simulink model "BlocoHidraulico"  (R2025a)
settings: Solver=ode15s  StartTime=0.0  StopTime=4  MaxStep=1e-4  RelTol=1e-3
values from neighbouring files (symbols this model uses):
  Pret = 1e5    (= 100000)    [ensaio_integrado_malha_aberta_real.m]    (also in ensaio_malha_fechada_lqi.m)
  Psup0 = Pret    (= 100000)    [ensaio_integrado_malha_aberta_real.m]
  Pw0 = Pret    (= 100000)    [ensaio_integrado_malha_aberta_real.m]
settings Model: Creator=uidq5744  LastModifiedBy=uidq5744

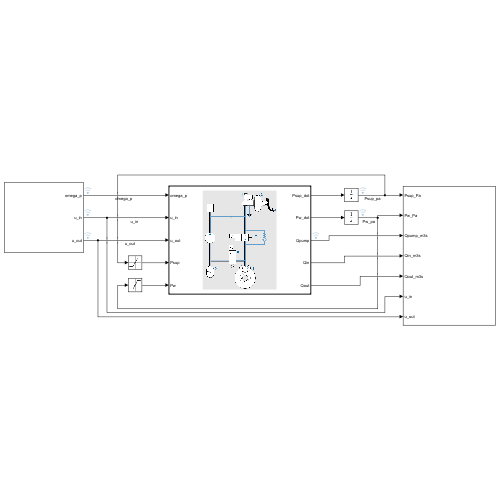
[thumbnail: Simulink's stored preview of the top-level diagram]
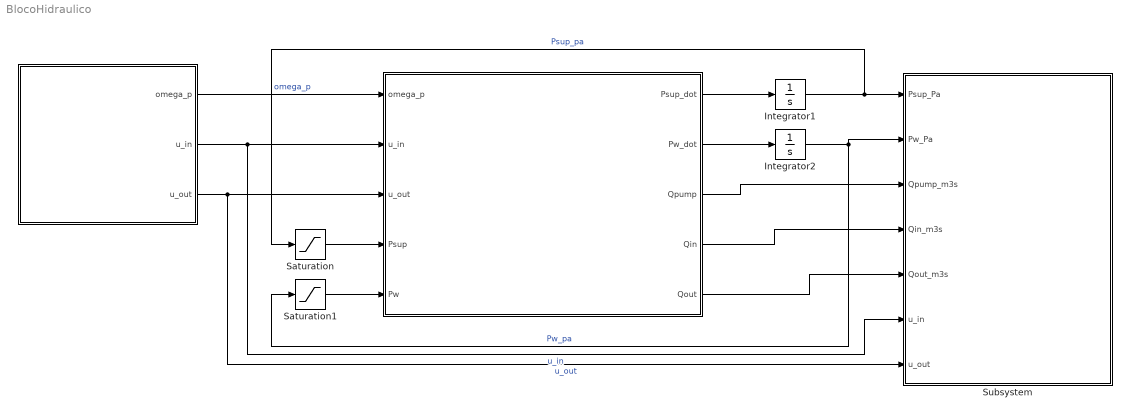
== system BlocoHidraulico ==
  " " : Subsystem
  "  " : MATLAB Function  TreatAsAtomicUnit=on
  Integrator1 : Integrator  InitialCondition=Psup0
  Integrator2 : Integrator  InitialCondition=Pw0
  Saturation : Saturate  UpperLimit=2.5e7  LowerLimit=Pret
  Saturation1 : Saturate  UpperLimit=2.5e7  LowerLimit=Pret
  Subsystem : Subsystem
  wires:
  Integrator1/1 -> Saturation/1, Subsystem/1(Psup_Pa)  "Psup_pa"
  " "/1(omega_p) -> "  "/1(omega_p)  "omega_p"
  " "/2(u_in) -> "  "/2(u_in), Subsystem/6(u_in)  "u_in"
  " "/3(u_out) -> "  "/3(u_out), Subsystem/7(u_out)  "u_out"
  "  "/1(Psup_dot) -> Integrator1/1
  "  "/2(Pw_dot) -> Integrator2/1
  Integrator2/1 -> Saturation1/1, Subsystem/2(Pw_Pa)  "Pw_pa"
  Saturation/1 -> "  "/4(Psup)
  Saturation1/1 -> "  "/5(Pw)
  "  "/3(Qpump) -> Subsystem/3(Qpump_m3s)
  "  "/4(Qin) -> Subsystem/4(Qin_m3s)
  "  "/5(Qout) -> Subsystem/5(Qout_m3s)

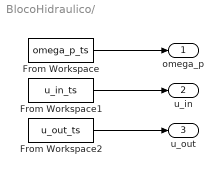
== system BlocoHidraulico/  ==
  From Workspace : FromWorkspace  VariableName=omega_p_ts
  From Workspace1 : FromWorkspace  VariableName=u_in_ts
  From Workspace2 : FromWorkspace  VariableName=u_out_ts
  omega_p : Outport
  u_in : Outport  Port=2
  u_out : Outport  Port=3
  wires:
  From Workspace/1 -> omega_p/1
  From Workspace1/1 -> u_in/1
  From Workspace2/1 -> u_out/1

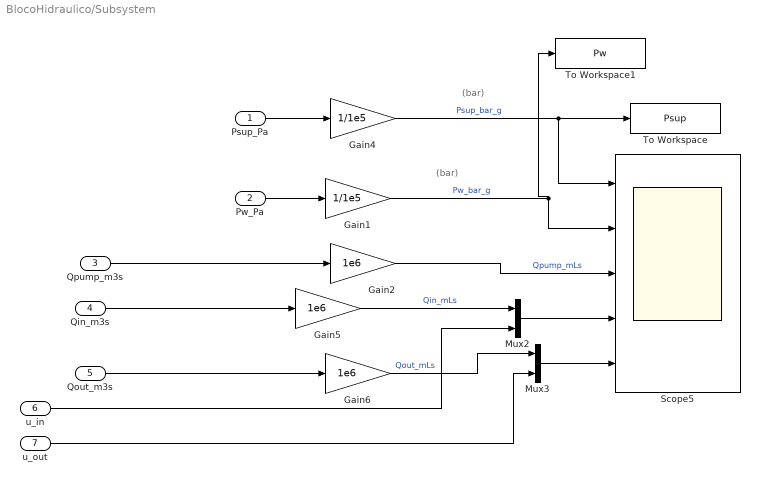
== system BlocoHidraulico/Subsystem ==
  note: (bar)
  note: (bar)
  Psup_Pa : Inport
  Pw_Pa : Inport  Port=2
  Qpump_m3s : Inport  Port=3
  Qin_m3s : Inport  Port=4
  Qout_m3s : Inport  Port=5
  u_in : Inport  Port=6
  u_out : Inport  Port=7
  Gain1 : Gain  Gain=1/1e5
  Gain2 : Gain  Gain=1e6
  Gain4 : Gain  Gain=1/1e5
  Gain5 : Gain  Gain=1e6
  Gain6 : Gain  Gain=1e6
  Mux2 : Mux  Inputs=2
  Mux3 : Mux  Inputs=2
  Scope5 : Scope  NumInputPorts=5
      settings: ActiveDisplayYMinimum=-13.920770076157355  ActiveDisplayYMaximum=135.28693068541622  DataLoggingVariableName=ScopeData6
  To Workspace : ToWorkspace  VariableName=Psup  SaveFormat=Timeseries  SampleTime=-1
  To Workspace1 : ToWorkspace  VariableName=Pw  SaveFormat=Timeseries  SampleTime=-1
  wires:
  Gain1/1 -> Scope5/2, To Workspace1/1  "Pw_bar_g"
  Mux2/1 -> Scope5/4
  Gain5/1 -> Mux2/1  "Qin_mLs"
  u_in/1 -> Mux2/2
  Gain2/1 -> Scope5/3  "Qpump_mLs"
  Gain4/1 -> Scope5/1, To Workspace/1  "Psup_bar_g"
  Gain6/1 -> Mux3/1  "Qout_mLs"
  Mux3/1 -> Scope5/5
  Psup_Pa/1 -> Gain4/1
  Qpump_m3s/1 -> Gain2/1
  Qout_m3s/1 -> Gain6/1
  Qin_m3s/1 -> Gain5/1
  u_out/1 -> Mux3/2
  Pw_Pa/1 -> Gain1/1

== matlab function BlocoHidraulico/   ==
  data: omega_p input; Psup_dot output; u_in input; u_out input; Psup input; Pw input; Pw_dot output; Qpump output; Qin output; Qout output
function [Psup_dot, Pw_dot, Qpump, Qin, Qout] = Bloco_Hidraulico_2P(omega_p, u_in, u_out, Psup, Pw)
% omega_p: rad/s (>=0)
% u_in, u_out: 0..1 (PWM normalizado / abertura proporcional)
% Psup, Pw: Pa
% Saídas: derivadas de pressão e vazões (m^3/s)

% ---------- parâmetros hidráulicos básicos ----------
beta = 1.5e9;   % Pa - módulo volumétrico efetivo (óleo + mangueiras)
rho  = 850;     % kg/m^3 - densidade típica de fluido de freio
Pret = 1e5;     % Pa - pressão de retorno (aprox. atmosférica)

% ---------- volumes efetivos ----------
% Ordens de grandeza compatíveis com circuitos de freio/HCU:
% - Lv2014, ChenLv2017: pequenas câmaras, respostas de 80–300 MPa/s.
%
% Vsup: volume efetivo do manifold/suprimento (linha de alta + câmara da HCU)
% Vw  : volume efetivo do circuito "roda"/caliper (câmara da pinça + linha)
Vsup = 6.0e-5;   % m^3  (~100 mL)
Vw   = 1.0e-5;   % m^3  (~10 mL)

% ---------- bomba (modelo linear simples) ----------
% Referência: bombas de HCU/IEB com deslocamentos da ordem de 0.1–1 cm^3/volta,
% vazões < 1 L/min em regimes típicos (WangBingbing2015, MotorParametricDesign2023).
%
Dp_rev = 5e-7;           % m^3/rev (0.5 cm^3/1000 rev; pequeno deslocamento por volta)
Nv     = 0.85;           % eficiência volumétrica
Kb     = Nv * (Dp_rev/(2*pi));   % m^3/rad  (Qpump = Kb*omega_p)
Klb    = 6.8e-13;          % (m^3/s)/Pa - vazamento interno equivalente (3e-13 a 8e-13)
% Klb (vazamento/bypass interno “de verdade”): 1e-14 a 5e-13 (ordem menor que hoje)

% ---------- válvulas (lei do orifício) ----------
% Coerente com diâmetros de ~0.6–0.8 mm (ChenLv2017, ProportionalPressureABS2023):
% A = pi*(d/2)^2. Para d ≈ 0.7 mm -> A ≈ 3.8e-7 m^2.
% Usamos área máxima ligeiramente menor para representar abertura efetiva.
Cv_in   = 0.62;          % coeficiente de descarga típico
Cv_out  = 0.62;
Ain_max = 3.0e-7;        % m^2 - área máx. da válvula de entrada
Aout_max= 3.0e-7;        % m^2 - área máx. da válvula de saída

% Vazamentos opcionais (para estabilidade numérica / perdas pequenas)
Kleak_sup = 0;           % (m^3/s)/Pa
Kleak_w   = 0;           % (m^3/s)/Pa

% ---------- sanitização de entradas ----------
if omega_p < 0
    omega_p = 0;
end
u_in  = min(max(u_in,  0), 1);
u_out = min(max(u_out, 0), 1);

% Evita pressões abaixo do retorno (numérico)
Psup = max(Psup, Pret);
Pw   = max(Pw,   Pret);

% ---------- bomba -> suprimento ----------
Qpump = Kb*omega_p - Klb*(Psup - Pret);
% Nota: usa (Psup - Pret) para não "puxar" abaixo da pressão de retorno.

% ---------- suprimento -> roda (válvula de entrada) ----------
dPin = max(Psup - Pw, 0);
Qin  = Cv_in * (Ain_max * u_in) * sqrt(2*dPin/rho);

% ---------- roda -> retorno (válvula de saída) ----------
dPout = max(Pw - Pret, 0);
Qout  = Cv_out * (Aout_max * u_out) * sqrt(2*dPout/rho);

% ---------- dinâmica das pressões ----------
Psup_dot = (beta/Vsup) * ( Qpump - Qin - Kleak_sup*(Psup - Pret) );
Pw_dot   = (beta/Vw)   * ( Qin - Qout - Kleak_w*(Pw   - Pret) );
end

%%
% β e ρ mantidos (compatíveis com Lv2014, MotorParametricDesign2023).
% Volumes Vsup, Vw ajustados para ordens de 10⁻⁶–10⁻⁷ m³ (câmara pequena de HCU e cilindro de roda) coerentes com Lv2014 / ChenLv2017 / ZengYangHuang2023.
% Bomba dimensionada para vazões ~0.5–1 L/min em faixas de rpm típicas de bomba ESC (coerente com MotorParametricDesign2023 e WangBingbing2015).
% Áreas de válvulas baseadas em diâmetros ~0.6–0.8 mm (ProportionalPressureABS2023, ChenLv2017).

% Com Vsup ≈ 2 mL e Vw ≈ 0.5 mL, beta/V fica na ordem de 10¹⁴–10¹⁵ s⁻¹·m⁻³, o que, combinado com vazões de ~10⁻⁶–10⁻⁵ m³/s, gera dP/dt na faixa de dezenas a poucas centenas de MPa/s – alinhado com os ~88.8 MPa/s (subida) e ~324.9 MPa/s (descida) medidos em ZengYangHuang2023.
% As áreas de válvula (~3e-7 m²) correspondem a diâmetros ~0.6–0.7 mm, compatíveis com os assentos/agulhas dos artigos ChenLv2017 e ProportionalPressureABS2023.
% O deslocamento da bomba (5e-7 m³/rev) é conservador, mas suficiente para gerar pressões de alguns MPa em tempos da ordem de 0.1–0.2 s para testes de malha aberta.


% function [Psup_dot, Pw_dot, Qpump, Qin, Qout] = Bloco_Hidraulico_2P(omega_p, u_in, u_out, Psup, Pw)
% % omega_p: rad/s (>=0)
% % u_in, u_out: 0..1 (PWM normalizado)
% % Psup, Pw: Pa
% % Saídas: derivadas de pressão e vazões (m^3/s)
% 
% % ---------- parâmetros ----------
% beta   = 1.5e9;      % Pa (módulo volumétrico efetivo)
% rho    = 850;        % kg/m^3
% Pret   = 1e5;        % Pa (reservatório/retorno)
% 
% % Volume teorico
% % Vsup   = 2.0e-5;     % m^3  (volume efetivo do manifold/suprimento) AJUSTAR
% % Vw     = 1.0e-5;     % m^3  (volume efetivo do circuito "roda"/caliper) AJUSTAR
% 
% % Volumes reduzidos (faixa de pressao mais alta)
% Vsup   = 5.0e-7;     % m^3  (volume efetivo do manifold/suprimento)
% Vw     = 5.0e-8;     % m^3  (volume efetivo do circuito "roda"/caliper)
% 
% % % Bomba (modelo linear simples)
% % Dp_rev = 1e-6;       % m^3/rev
% % Nv  = 0.85;       % Eficiência volumétrica da bomba
% % Kb     = Nv*(Dp_rev/(2*pi)); % m^3/rad
% % Klb    = 1e-10;      % (m^3/s)/Pa  (vazamento interno equivalente)
% 
% % Bomba (parâmetros ajustados)
% Dp_rev = 1e-5;       % m^3/rev (deslocamento volumétrico por volta)
% Nv     = 0.85;       % Eficiência volumétrica da bomba
% Kb     = Nv*(Dp_rev/(2*pi)); % m^3/rad
% Klb    = 1e-11;      % (m^3/s)/Pa  (vazamento interno equivalente)
% 
% % Válvulas (lei do orifício)
% Cv_in   = 0.62;
% Cv_out  = 0.62;
% Ain_max = 1e-7;      % m^2
% Aout_max= 1e-7;      % m^2
% 
% Kleak_sup = 0;       % (m^3/s)/Pa opcional
% Kleak_w   = 0;       % (m^3/s)/Pa opcional
% 
% % ---------- sanitização ----------
% if omega_p < 0, omega_p = 0; end
% u_in  = min(max(u_in, 0), 1);
% u_out = min(max(u_out,0), 1);
% 
% % Evita pressões abaixo do retorno (numérico)
% Psup = max(Psup, Pret);
% Pw   = max(Pw,   Pret);
% 
% % ---------- bomba -> suprimento ----------
% Qpump = Kb*omega_p - Klb*(Psup - Pret);
% % Observação: use (Psup-Pret) aqui pra não "puxar" abaixo de Pret.
% 
% % ---------- suprimento -> roda (válvula de entrada) ----------
% dPin = max(Psup - Pw, 0);
% Qin  = Cv_in*(Ain_max*u_in)*sqrt(2*dPin/rho);
% 
% % ---------- roda -> retorno (válvula de saída) ----------
% dPout = max(Pw - Pret, 0);
% Qout  = Cv_out*(Aout_max*u_out)*sqrt(2*dPout/rho);
% 
% % ---------- dinâmica das pressões ----------
% Psup_dot = (beta/Vsup)*( Qpump - Qin - Kleak_sup*(Psup-Pret) );
% Pw_dot   = (beta/Vw)  *( Qin - Qout - Kleak_w*(Pw-Pret) );
% end
